simulink model "DYN_03"  (R2021a)
settings: Solver=FixedStepAuto  StartTime=0.0  StopTime=50  FixedStep=0.001  RelTol=1e-3
settings Model: Creator=TMP  LastModifiedBy=TMP
settings SolverCC: AlgebraicLoopSolver=TrustRegion
settings DebuggingCC: SFMachineParentedDataDiag=warning

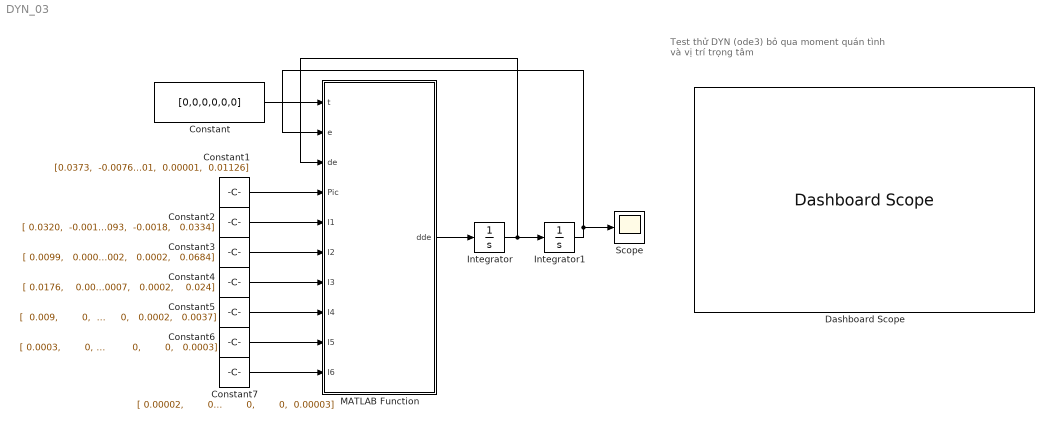
== system DYN_03 ==
  note: Test thử DYN (ode3)
      | bỏ qua moment quán tình và vị trí trọng tâm
  Constant : Constant  Value=[0,0,0,0,0,0]
  Constant1 : Constant  Value=|
      | [0.0373,  -0.0076,   0.1064;
      |        0.1127,   0.0065,   0.0648;
      |        0.0447,   0.0125,  -0.0554;
      |        0.0006,   0.0052,   0.1068;
      |             0,   0.0062,   0.0195;
      |      -0.00001,  0.00001,  0.01126]
  Constant2 : Constant  Value=|
      | [ 0.0320,  -0.0017,   0.0093;
      |       -0.0017,   0.0364,  -0.0018;
      |        0.0093,  -0.0018,   0.0334]
  Constant3 : Constant  Value=|
      | [ 0.0099,   0.0008,  -0.0002;
      |        0.0008,   0.0646,   0.0002;
      |       -0.0002,   0.0002,   0.0684]
  Constant4 : Constant  Value=|
      | [ 0.0176,    0.001,   0.0007;
      |         0.001,   0.0195,   0.0002;
      |        0.0007,   0.0002,    0.024]
  Constant5 : Constant  Value=|
      | [  0.009,        0,        0;
      |             0,   0.0081,   0.0002;
      |             0,   0.0002,   0.0037]
  Constant6 : Constant  Value=|
      | [ 0.0003,        0,        0;
      |             0,   0.0002,        0;
      |             0,        0,   0.0003]
  Constant7 : Constant  Value=|
      | [ 0.00002,        0,        0;
      |              0,  0.00002,        0;
      |              0,        0,  0.00003]
  Dashboard Scope : DashboardScope
  Integrator : Integrator  InitialCondition=[0.2;0.2;0.2;0.2;0.2;0.2]
  Integrator1 : Integrator  InitialCondition=[0.1;0.1;0.1;0.1;0.1;0.1]
  MATLAB Function : MATLAB Function  TreatAsAtomicUnit=on
  Scope : Scope
  wires:
  MATLAB Function/1(dde) -> Integrator/1
  Integrator/1 -> MATLAB Function/3(de), Integrator1/1
  Integrator1/1 -> MATLAB Function/2(e), Scope/1
  Constant/1 -> MATLAB Function/1(t)
  Constant1/1 -> MATLAB Function/4(Pic)
  Constant2/1 -> MATLAB Function/5(I1)
  Constant3/1 -> MATLAB Function/6(I2)
  Constant4/1 -> MATLAB Function/7(I3)
  Constant5/1 -> MATLAB Function/8(I4)
  Constant6/1 -> MATLAB Function/9(I5)
  Constant7/1 -> MATLAB Function/10(I6)

== matlab function DYN_03/MATLAB Function ==
  data: t input; e input; dde output; de input; Pic input; I1 input; I2 input; I3 input; I4 input; I5 input; I6 input
function dde = fcn(t,e,de,Pic,I1,I2,I3,I4,I5,I6)
e1 = e(1); e2 = e(2); e3 = e(3);
e4 = e(4); e5 = e(5); e6 = e(6);
de1 = de(1); de2 = de(2); de3 = de(3);
de4 = de(4); de5 = de(5); de6 = de(6);
x1 = Pic(1,1); y1 = Pic(1,2); z1 = Pic(1,3);
x2 = Pic(2,1); y2 = Pic(2,2); z2 = Pic(2,3);
x3 = Pic(3,1); y3 = Pic(3,2); z3 = Pic(3,3);
x4 = Pic(4,1); y4 = Pic(4,2); z4 = Pic(4,3);
x5 = Pic(5,1); y5 = Pic(5,2); z5 = Pic(5,3);
x6 = Pic(6,1); y6 = Pic(6,2); z6 = Pic(6,3);
I1xx = I1(1,1); I1xy = I1(1,2); I1xz = I1(1,3);
I1yx = I1(2,1); I1yy = I1(2,2); I1yz = I1(2,3);
I1zx = I1(3,1); I1zy = I1(3,2); I1zz = I1(3,3);

I2xx = I2(1,1); I2xy = I2(1,2); I2xz = I2(1,3);
I2yx = I2(2,1); I2yy = I2(2,2); I2yz = I2(2,3);
I2zx = I2(3,1); I2zy = I2(3,2); I2zz = I2(3,3);

I3xx = I3(1,1); I3xy = I3(1,2); I3xz = I3(1,3);
I3yx = I3(2,1); I3yy = I3(2,2); I3yz = I3(2,3);
I3zx = I3(3,1); I3zy = I3(3,2); I3zz = I3(3,3);

I4xx = I4(1,1); I4xy = I4(1,2); I4xz = I4(1,3);
I4yx = I4(2,1); I4yy = I4(2,2); I4yz = I4(2,3);
I4zx = I4(3,1); I4zy = I4(3,2); I4zz = I4(3,3);

I5xx = I5(1,1); I5xy = I5(1,2); I5xz = I5(1,3);
I5yx = I5(2,1); I5yy = I5(2,2); I5yz = I5(2,3);
I5zx = I5(3,1); I5zy = I5(3,2); I5zz = I5(3,3);

I6xx = I6(1,1); I6xy = I6(1,2); I6xz = I6(1,3);
I6yx = I6(2,1); I6yy = I6(2,2); I6yz = I6(2,3);
I6zx = I6(3,1); I6zy = I6(3,2); I6zz = I6(3,3);
a1=0.75; a2=2.70; a3=0.90; d1=3.35; d4=2.95; d7=0.80;
m0 = 7.2407; m1 = 5.6511; m2 = 4.6061; m3 = 4.2963; m4 = 1.9151; m5 = 0.3399; m6 = 0.0714;
g = 9.80665;
%% 

J = ...
[ d4*sin(e1)*sin(e2)*sin(e3) - a2*sin(e1)*sin(e2) - d4*cos(e2)*cos(e3)*sin(e1) - a3*cos(e2)*sin(e1)*sin(e3) - a3*cos(e3)*sin(e1)*sin(e2) - d7*cos(e1)*sin(e4)*sin(e5) - a1*sin(e1) - d7*cos(e2)*cos(e3)*cos(e5)*sin(e1) + d7*cos(e5)*sin(e1)*sin(e2)*sin(e3) + d7*cos(e2)*cos(e4)*sin(e1)*sin(e3)*sin(e5) + d7*cos(e3)*cos(e4)*sin(e1)*sin(e2)*sin(e5), -cos(e1)*(d4*cos(e2)*sin(e3) - a3*cos(e2)*cos(e3) - a2*cos(e2) + d4*cos(e3)*sin(e2) + a3*sin(e2)*sin(e3) + d7*cos(e2)*cos(e5)*sin(e3) + d7*cos(e3)*cos(e5)*sin(e2) + d7*cos(e2)*cos(e3)*cos(e4)*sin(e5) - d7*cos(e4)*sin(e2)*sin(e3)*sin(e5)), -cos(e1)*(d4*cos(e2)*sin(e3) - a3*cos(e2)*cos(e3) + d4*cos(e3)*sin(e2) + a3*sin(e2)*sin(e3) + d7*cos(e2)*cos(e5)*sin(e3) + d7*cos(e3)*cos(e5)*sin(e2) + d7*cos(e2)*cos(e3)*cos(e4)*sin(e5) - d7*cos(e4)*sin(e2)*sin(e3)*sin(e5)), d7*sin(e5)*(cos(e1)*cos(e2)*sin(e3)*sin(e4) - cos(e4)*sin(e1) + cos(e1)*cos(e3)*sin(e2)*sin(e4)), d7*cos(e1)*sin(e2)*sin(e3)*sin(e5) - d7*cos(e1)*cos(e2)*cos(e3)*sin(e5) - d7*cos(e5)*sin(e1)*sin(e4) - d7*cos(e1)*cos(e2)*cos(e4)*cos(e5)*sin(e3) - d7*cos(e1)*cos(e3)*cos(e4)*cos(e5)*sin(e2),                                                                                                                            0;
  a1*cos(e1) + a2*cos(e1)*sin(e2) + d4*cos(e1)*cos(e2)*cos(e3) + a3*cos(e1)*cos(e2)*sin(e3) + a3*cos(e1)*cos(e3)*sin(e2) - d4*cos(e1)*sin(e2)*sin(e3) - d7*sin(e1)*sin(e4)*sin(e5) + d7*cos(e1)*cos(e2)*cos(e3)*cos(e5) - d7*cos(e1)*cos(e5)*sin(e2)*sin(e3) - d7*cos(e1)*cos(e2)*cos(e4)*sin(e3)*sin(e5) - d7*cos(e1)*cos(e3)*cos(e4)*sin(e2)*sin(e5), -sin(e1)*(d4*cos(e2)*sin(e3) - a3*cos(e2)*cos(e3) - a2*cos(e2) + d4*cos(e3)*sin(e2) + a3*sin(e2)*sin(e3) + d7*cos(e2)*cos(e5)*sin(e3) + d7*cos(e3)*cos(e5)*sin(e2) + d7*cos(e2)*cos(e3)*cos(e4)*sin(e5) - d7*cos(e4)*sin(e2)*sin(e3)*sin(e5)), -sin(e1)*(d4*cos(e2)*sin(e3) - a3*cos(e2)*cos(e3) + d4*cos(e3)*sin(e2) + a3*sin(e2)*sin(e3) + d7*cos(e2)*cos(e5)*sin(e3) + d7*cos(e3)*cos(e5)*sin(e2) + d7*cos(e2)*cos(e3)*cos(e4)*sin(e5) - d7*cos(e4)*sin(e2)*sin(e3)*sin(e5)), d7*sin(e5)*(cos(e1)*cos(e4) + cos(e2)*sin(e1)*sin(e3)*sin(e4) + cos(e3)*sin(e1)*sin(e2)*sin(e4)), d7*cos(e1)*cos(e5)*sin(e4) - d7*cos(e2)*cos(e3)*sin(e1)*sin(e5) + d7*sin(e1)*sin(e2)*sin(e3)*sin(e5) - d7*cos(e2)*cos(e4)*cos(e5)*sin(e1)*sin(e3) - d7*cos(e3)*cos(e4)*cos(e5)*sin(e1)*sin(e2),                                                                                                                            0;
                                                                                                                                                                                                                                                                                                                                                     0,            d4*sin(e2)*sin(e3) - d4*cos(e2)*cos(e3) - a3*cos(e2)*sin(e3) - a3*cos(e3)*sin(e2) - a2*sin(e2) - d7*cos(e2)*cos(e3)*cos(e5) + d7*cos(e5)*sin(e2)*sin(e3) + d7*cos(e2)*cos(e4)*sin(e3)*sin(e5) + d7*cos(e3)*cos(e4)*sin(e2)*sin(e5),            d4*sin(e2)*sin(e3) - a3*cos(e2)*sin(e3) - a3*cos(e3)*sin(e2) - d4*cos(e2)*cos(e3) - d7*cos(e2)*cos(e3)*cos(e5) + d7*cos(e5)*sin(e2)*sin(e3) + d7*cos(e2)*cos(e4)*sin(e3)*sin(e5) + d7*cos(e3)*cos(e4)*sin(e2)*sin(e5),                                                                  d7*cos(e2 + e3)*sin(e4)*sin(e5),                                                              d7*cos(e2)*sin(e3)*sin(e5) + d7*cos(e3)*sin(e2)*sin(e5) - d7*cos(e2)*cos(e3)*cos(e4)*cos(e5) + d7*cos(e4)*cos(e5)*sin(e2)*sin(e3),                                                                                                                            0;
                                                                                                                                                                                                                                                                                                                                                     0,                                                                                                                                                                                                                                      -sin(e1),                                                                                                                                                                                                                         -sin(e1),                                                                             cos(e2 + e3)*cos(e1),                                                                                                            cos(e1)*cos(e2)*sin(e3)*sin(e4) - cos(e4)*sin(e1) + cos(e1)*cos(e3)*sin(e2)*sin(e4), cos(e2 + e3)*cos(e1)*cos(e5) - sin(e5)*(sin(e1)*sin(e4) + cos(e1)*cos(e2)*cos(e4)*sin(e3) + cos(e1)*cos(e3)*cos(e4)*sin(e2));
                                                                                                                                                                                                                                                                                                                                                     0,                                                                                                                                                                                                                                       cos(e1),                                                                                                                                                                                                                          cos(e1),                                                                             cos(e2 + e3)*sin(e1),                                                                                                            cos(e1)*cos(e4) + cos(e2)*sin(e1)*sin(e3)*sin(e4) + cos(e3)*sin(e1)*sin(e2)*sin(e4), cos(e2 + e3)*cos(e5)*sin(e1) - sin(e5)*(cos(e2)*cos(e4)*sin(e1)*sin(e3) - cos(e1)*sin(e4) + cos(e3)*cos(e4)*sin(e1)*sin(e2));                                                                                                                                                                                                                                                                                                                                                   1,                                                                                                                                                                                                                                             0,                                                                                                                                                                                                                                0,                                                                                    -sin(e2 + e3),                                                                                                                                                                           cos(e2 + e3)*sin(e4),                                                                        - sin(e2 + e3)*cos(e5) - cos(e2 + e3)*cos(e4)*sin(e5)];
%%
% V = [V1+5*dt1;V2+5*dt2;V3+5*dt3];
de = [de1;de2;de3;de4;de5;de6];
% V = C*de;
% M_inv = inv(M);
c = 0;
b = 0;
Fe = 0*[1;1;1;1;1;1];
F = c*sign(de) + b*de + J'*Fe ;
dde = M\(t-C*de-G-F);
